simulink model "DC_Grid_New"  (R2022b)
settings: Solver=FixedStepAuto  StartTime=0.0  StopTime=48  FixedStep=0.01  RelTol=1e-3
undefined symbols (not defined in the file): C, cableLV, cableMV, flexible_load_autumn_shifted, flexible_load_spring_shifted, flexible_load_summer_shifted, flexible_load_winter_shifted, LowLoadP, LV, MV, PeakShP, Scaling_factor, Wind_scalefactor
libraries: DC_GRIDSIM_LIB x80, simulink x12
settings Model: Creator=mingreico  LastModifiedBy=mingreico

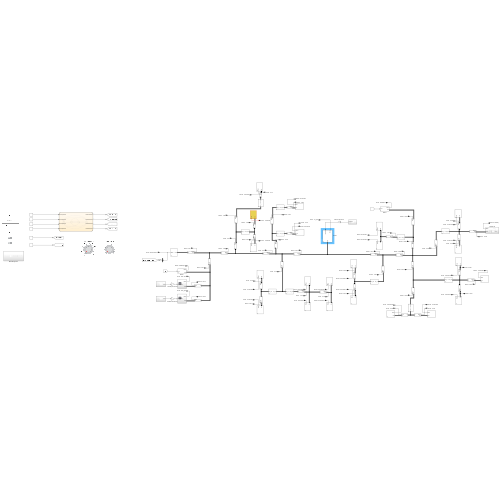
[thumbnail: Simulink's stored preview of the top-level diagram]
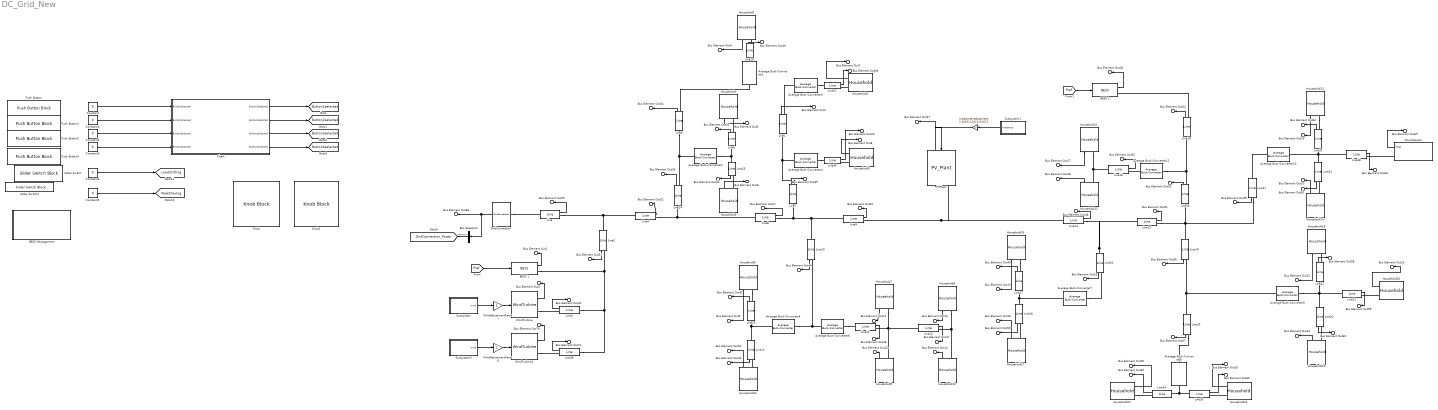
== system DC_Grid_New ==
  Average Buck-Converter{1..10,12} (11 alike) : DC_GRIDSIM_LIB/Average Buck-Converter  C=C  D=LV/MV
      settings: SourceProductName=DC GRIDSIM Library
  BESS 1 : DC_GRIDSIM_LIB/BESS  V_Bat=MV  Qbat=10000  SOC_init=0.5  SOC_min=0.1  SOC_max=0.9  P_max=10000
      settings: SourceProductName=DC GRIDSIM Library
  BESS 2 : DC_GRIDSIM_LIB/BESS  V_Bat=MV  Qbat=10000  SOC_init=0.5  SOC_min=0.1  SOC_max=0.9  P_max=10000
      settings: SourceProductName=DC GRIDSIM Library
  BESS Management : Subsystem
  Bus Selector2 : BusSelector  OutputSignals=Power
  Chart : Stateflow chart  TreatAsAtomicUnit=on
  Constant{,1..3} (4 alike) : Constant  Value=0  OutDataTypeStr=boolean
  Constant4 : Constant  Value=0
  Constant5 : Constant  Value=0
  FlexibleLoad : Subsystem
  GridConnection : DC_GRIDSIM_LIB/GridConnection  MV_Ref=MV
      settings: SourceProductName=DC GRIDSIM Library
  Household1 : DC_GRIDSIM_LIB/Household  ProfileSpring=Household4_Springallday  ProfileSummer=Household4_Summerallday  ProfileAutumn=Household4_Autumnallday  ProfileWinter=Household4_Winterallday  Timevector=Allday_timevector  k=Scaling_factor  VnomLoad=LV
      settings: SourceProductName=DC GRIDSIM Library
  Household10 : DC_GRIDSIM_LIB/Household  ProfileSpring=Household15_Springallday  ProfileSummer=Household15_Summerallday  ProfileAutumn=Household15_Autumnallday  ProfileWinter=Household15_Winterallday  Timevector=Allday_timevector  k=Scaling_factor  VnomLoad=LV
      settings: SourceProductName=DC GRIDSIM Library
  Household11 : DC_GRIDSIM_LIB/Household  ProfileSpring=Household26_Springallday  ProfileSummer=Household26_Summerallday  ProfileAutumn=Household26_Autumnallday  ProfileWinter=Household26_Winterallday  Timevector=Allday_timevector  k=Scaling_factor  VnomLoad=LV
      settings: SourceProductName=DC GRIDSIM Library
  Household12 : DC_GRIDSIM_LIB/Household  ProfileSpring=Household8_Springallday  ProfileSummer=Household8_Summerallday  ProfileAutumn=Household8_Autumnallday  ProfileWinter=Household8_Winterallday  Timevector=Allday_timevector  k=Scaling_factor  VnomLoad=LV
      settings: SourceProductName=DC GRIDSIM Library
  Household13 : DC_GRIDSIM_LIB/Household  ProfileSpring=Household9_Springallday  ProfileSummer=Household9_Summerallday  ProfileAutumn=Household9_Autumnallday  ProfileWinter=Household9_Winterallday  Timevector=Allday_timevector  k=Scaling_factor  VnomLoad=LV
      settings: SourceProductName=DC GRIDSIM Library
  Household14 : DC_GRIDSIM_LIB/Household  ProfileSpring=Household12_Springallday  ProfileSummer=Household12_Summerallday  ProfileAutumn=Household12_Autumnallday  ProfileWinter=Household12_Winterallday  Timevector=Allday_timevector  k=Scaling_factor  VnomLoad=LV
      settings: SourceProductName=DC GRIDSIM Library
  Household16 : DC_GRIDSIM_LIB/Household  ProfileSpring=Household11_Springallday  ProfileSummer=Household11_Summerallday  ProfileAutumn=Household11_Autumnallday  ProfileWinter=Household11_Winterallday  Timevector=Allday_timevector  k=Scaling_factor  VnomLoad=LV
      settings: SourceProductName=DC GRIDSIM Library
  Household17 : DC_GRIDSIM_LIB/Household  ProfileSpring=Household12_Springallday  ProfileSummer=Household12_Summerallday  ProfileAutumn=Household12_Autumnallday  ProfileWinter=Household12_Winterallday  Timevector=Allday_timevector  k=Scaling_factor  VnomLoad=LV
      settings: SourceProductName=DC GRIDSIM Library
  Household18 : DC_GRIDSIM_LIB/Household  ProfileSpring=Household3_Springallday  ProfileSummer=Household3_Summerallday  ProfileAutumn=Household3_Autumnallday  ProfileWinter=Household3_Winterallday  Timevector=Allday_timevector  k=Scaling_factor  VnomLoad=LV
      settings: SourceProductName=DC GRIDSIM Library
  Household19 : DC_GRIDSIM_LIB/Household  ProfileSpring=Household7_Springallday  ProfileSummer=Household7_Summerallday  ProfileAutumn=Household7_Autumnallday  ProfileWinter=Household7_Winterallday  Timevector=Allday_timevector  k=Scaling_factor  VnomLoad=LV
      settings: SourceProductName=DC GRIDSIM Library
  Household2 : DC_GRIDSIM_LIB/Household  ProfileSpring=Household3_Springallday  ProfileSummer=Household3_Summerallday  ProfileAutumn=Household3_Autumnallday  ProfileWinter=Household3_Winterallday  Timevector=Allday_timevector  k=Scaling_factor  VnomLoad=LV
      settings: SourceProductName=DC GRIDSIM Library
  Household20 : DC_GRIDSIM_LIB/Household  ProfileSpring=Household8_Springallday  ProfileSummer=Household8_Summerallday  ProfileAutumn=Household8_Autumnallday  ProfileWinter=Household8_Winterallday  Timevector=Allday_timevector  k=Scaling_factor  VnomLoad=LV
      settings: SourceProductName=DC GRIDSIM Library
  Household21 : DC_GRIDSIM_LIB/Household  ProfileSpring=Household10_Springallday  ProfileSummer=Household10_Summerallday  ProfileAutumn=Household10_Autumnallday  ProfileWinter=Household10_Winterallday  Timevector=Allday_timevector  k=Scaling_factor  VnomLoad=LV
      settings: SourceProductName=DC GRIDSIM Library
  Household22 : DC_GRIDSIM_LIB/Household  ProfileSpring=Household26_Springallday  ProfileSummer=Household26_Summerallday  ProfileAutumn=Household26_Autumnallday  ProfileWinter=Household26_Winterallday  Timevector=Allday_timevector  k=Scaling_factor  VnomLoad=LV
      settings: SourceProductName=DC GRIDSIM Library
  Household23 : DC_GRIDSIM_LIB/Household  ProfileSpring=Household33_Springallday  ProfileSummer=Household33_Summerallday  ProfileAutumn=Household33_Autumnallday  ProfileWinter=Household33_Winterallday  Timevector=Allday_timevector  k=Scaling_factor  VnomLoad=LV
      settings: SourceProductName=DC GRIDSIM Library
  Household3 : DC_GRIDSIM_LIB/Household  ProfileSpring=Household5_Springallday  ProfileSummer=Household5_Summerallday  ProfileAutumn=Household5_Autumnallday  ProfileWinter=Household5_Winterallday  Timevector=Allday_timevector  k=Scaling_factor  VnomLoad=LV
      settings: SourceProductName=DC GRIDSIM Library
  Household4 : DC_GRIDSIM_LIB/Household  ProfileSpring=Household7_Springallday  ProfileSummer=Household7_Summerallday  ProfileAutumn=Household7_Autumnallday  ProfileWinter=Household7_Winterallday  Timevector=Allday_timevector  k=Scaling_factor  VnomLoad=LV
      settings: SourceProductName=DC GRIDSIM Library
  Household5 : DC_GRIDSIM_LIB/Household  ProfileSpring=Household8_Springallday  ProfileSummer=Household8_Summerallday  ProfileAutumn=Household8_Autumnallday  ProfileWinter=Household8_Winterallday  Timevector=Allday_timevector  k=Scaling_factor  VnomLoad=LV
      settings: SourceProductName=DC GRIDSIM Library
  Household6 : DC_GRIDSIM_LIB/Household  ProfileSpring=Household9_Springallday  ProfileSummer=Household9_Summerallday  ProfileAutumn=Household9_Autumnallday  ProfileWinter=Household9_Winterallday  Timevector=Allday_timevector  k=Scaling_factor  VnomLoad=LV
      settings: SourceProductName=DC GRIDSIM Library
  Household7 : DC_GRIDSIM_LIB/Household  ProfileSpring=Household11_Springallday  ProfileSummer=Household11_Summerallday  ProfileAutumn=Household11_Autumnallday  ProfileWinter=Household11_Winterallday  Timevector=Allday_timevector  k=Scaling_factor  VnomLoad=LV
      settings: SourceProductName=DC GRIDSIM Library
  Household8 : DC_GRIDSIM_LIB/Household  ProfileSpring=Household14_Springallday  ProfileSummer=Household14_Summerallday  ProfileAutumn=Household14_Autumnallday  ProfileWinter=Household14_Winterallday  Timevector=Allday_timevector  k=Scaling_factor  VnomLoad=LV
      settings: SourceProductName=DC GRIDSIM Library
  Household9 : DC_GRIDSIM_LIB/Household  ProfileSpring=Household12_Springallday  ProfileSummer=Household12_Summerallday  ProfileAutumn=Household12_Autumnallday  ProfileWinter=Household12_Winterallday  Timevector=Allday_timevector  k=Scaling_factor  VnomLoad=LV
      settings: SourceProductName=DC GRIDSIM Library
  "Irradiance-adjustment " : Gain  Gain=0.9883216814160616
  Knob : KnobBlock  ScaleMin=0.9  ScaleMax=3  TickInterval=0.1
  Knob1 : KnobBlock  ScaleMin=0.9  ScaleMax=3  TickInterval=0.1
  Line : DC_GRIDSIM_LIB/Line  rho=rhoMV  l=1.4e3  A=cableMV
      settings: SourceProductName=DC GRIDSIM Library
  Line{1,4,7,14} (4 alike) : DC_GRIDSIM_LIB/Line  rho=rhoMV  l=1.3e3  A=cableMV
      settings: SourceProductName=DC GRIDSIM Library
  Line{5,8,10,17,24,30} (6 alike) : DC_GRIDSIM_LIB/Line  rho=rhoMV  l=1e3  A=cableMV
      settings: SourceProductName=DC GRIDSIM Library
  Line{6,11,13,21,25,27,38} (7 alike) : DC_GRIDSIM_LIB/Line  rho=rhoLV  l=50  A=cableLV
      settings: SourceProductName=DC GRIDSIM Library
  Line{12,23,31,33,36} (5 alike) : DC_GRIDSIM_LIB/Line  rho=rhoLV  l=35  A=cableLV
      settings: SourceProductName=DC GRIDSIM Library
  Line15 : DC_GRIDSIM_LIB/Line  rho=rhoMV  l=0.5e3  A=cableMV
      settings: SourceProductName=DC GRIDSIM Library
  Line16 : DC_GRIDSIM_LIB/Line  rho=rhoLV  l=10  A=cableLV
      settings: SourceProductName=DC GRIDSIM Library
  Line18 : DC_GRIDSIM_LIB/Line  rho=rhoMV  l=1.2e3  A=cableMV
      settings: SourceProductName=DC GRIDSIM Library
  Line19 : DC_GRIDSIM_LIB/Line  rho=rhoMV  l=0.6e3  A=cableMV
      settings: SourceProductName=DC GRIDSIM Library
  Line2 : DC_GRIDSIM_LIB/Line  rho=rhoMV  l=0.3e3  A=cableMV
      settings: SourceProductName=DC GRIDSIM Library
  Line20 : DC_GRIDSIM_LIB/Line  rho=rhoLV  l=45  A=cableLV
      settings: SourceProductName=DC GRIDSIM Library
  Line22 : DC_GRIDSIM_LIB/Line  rho=rhoLV  l=45  A=cableLV
      settings: SourceProductName=DC GRIDSIM Library
  Line26 : DC_GRIDSIM_LIB/Line  rho=1.68e-8  l=1.0  A=240e-6
      settings: SourceProductName=DC GRIDSIM Library
  Line28 : DC_GRIDSIM_LIB/Line  rho=rhoLV  l=60  A=cableLV
      settings: SourceProductName=DC GRIDSIM Library
  Line29 : DC_GRIDSIM_LIB/Line  rho=rhoMV  l=0.4e3  A=cableMV
      settings: SourceProductName=DC GRIDSIM Library
  Line3 : DC_GRIDSIM_LIB/Line  rho=rhoMV  l=0.3e3  A=cableMV
      settings: SourceProductName=DC GRIDSIM Library
  Line32 : DC_GRIDSIM_LIB/Line  rho=rhoLV  l=0.5e3  A=cableLV
      settings: SourceProductName=DC GRIDSIM Library
  Line34 : DC_GRIDSIM_LIB/Line  rho=rhoLV  l=70  A=cableLV
      settings: SourceProductName=DC GRIDSIM Library
  Line35 : DC_GRIDSIM_LIB/Line  rho=rhoLV  l=70  A=cableLV
      settings: SourceProductName=DC GRIDSIM Library
  Line37 : DC_GRIDSIM_LIB/Line  rho=rhoLV  l=60  A=cableLV
      settings: SourceProductName=DC GRIDSIM Library
  Line39 : DC_GRIDSIM_LIB/Line  rho=rhoMV  l=0.3e3  A=cableMV
      settings: SourceProductName=DC GRIDSIM Library
  Line9 : DC_GRIDSIM_LIB/Line  rho=rhoMV  l=2e3  A=cableMV
      settings: SourceProductName=DC GRIDSIM Library
  PVPlant : DC_GRIDSIM_LIB/PV_Plant  f_tilt=1.1  P_mpp=260e3  PR=0.8
      settings: SourceProductName=DC GRIDSIM Library
  Push Button : PushButtonBlock  ButtonText=Button_SpringAllday  OffValue=0.000000
  Push Button1 : PushButtonBlock  ButtonText=Button_SummerAllday  OffValue=0.000000
  Push Button2 : PushButtonBlock  ButtonText=Button_AutumnAllday  OffValue=0.000000
  Push Button3 : PushButtonBlock  ButtonText=Button_WinterAllday  OffValue=0.000000
  Slider Switch : SliderSwitchBlock  LabelPosition=Hide
      settings: Values={{'NOShift', 'FlexibleLoad_Shifted'}, [0 1]}
  Slider Switch1 : SliderSwitchBlock  LabelPosition=Hide
      settings: Values={{'NoPeakShaving', 'Peakshaved'}, [0 1]}
  Subsystem : Subsystem
  Subsystem1 : Subsystem
  Subsystem2 : Subsystem
  WindAdjustmentFactor : Gain
  WindAdjustmentFactor1 : Gain
  WindTurbine : DC_GRIDSIM_LIB/WindTurbine  SystemSampleTime=-1  VariantActivationTime=update diagram  Latency=0  AutoFrameSizeCalculation=off
      link override Blade radius: Value=28
      settings: SourceProductName=DC GRIDSIM Library
  WindTurbine1 : DC_GRIDSIM_LIB/WindTurbine  SystemSampleTime=-1  VariantActivationTime=update diagram  Latency=0  AutoFrameSizeCalculation=off
      link override Blade radius: Value=28
      settings: SourceProductName=DC GRIDSIM Library
  Bus Element Out38 : Outport  PortName=Results  Element=GridConnection
  Bus Element Out1 : Outport  PortName=Results  Element=GridBattery1
  Bus Element Out2 : Outport  PortName=Results  Element=Wind_gen1
  Bus Element Out4 : Outport  PortName=Results  Element=Household1
  Bus Element Out5 : Outport  PortName=Results  Element=Household2
  Bus Element Out6 : Outport  PortName=Results  Element=Household3
  Bus Element Out7 : Outport  PortName=Results  Element=Household4
  Bus Element Out8 : Outport  PortName=Results  Element=Household5
  Bus Element Out9 : Outport  PortName=Results  Element=Household6
  Bus Element Out10 : Outport  PortName=Results  Element=Household7
  Bus Element Out11 : Outport  PortName=Results  Element=Household8
  Bus Element Out12 : Outport  PortName=Results  Element=Household9
  Bus Element Out13 : Outport  PortName=Results  Element=Household10
  Bus Element Out14 : Outport  PortName=Results  Element=Household11
  Bus Element Out15 : Outport  PortName=Results  Element=Household12
  Bus Element Out16 : Outport  PortName=Results  Element=Household13
  Bus Element Out17 : Outport  PortName=Results  Element=Household14
  Bus Element Out18 : Outport  PortName=Results  Element=Household15
  Bus Element Out19 : Outport  PortName=Results  Element=Household16
  Bus Element Out20 : Outport  PortName=Results  Element=Household17
  Bus Element Out22 : Outport  PortName=Results  Element=Household19
  Bus Element Out23 : Outport  PortName=Results  Element=Household20
  Bus Element Out24 : Outport  PortName=Results  Element=Household21
  Bus Element Out25 : Outport  PortName=Results  Element=Household22
  Bus Element Out26 : Outport  PortName=Results  Element=Household23
  Bus Element Out27 : Outport  PortName=Results  Element=PV_gen1
  Bus Element Out28 : Outport  PortName=Results  Element=GridBattery2
  Bus Element Out29 : Outport  PortName=Results  Element=Line1
  Bus Element Out31 : Outport  PortName=Results  Element=Line3
  Bus Element Out32 : Outport  PortName=Results  Element=Line4
  Bus Element Out33 : Outport  PortName=Results  Element=Line5
  Bus Element Out34 : Outport  PortName=Results  Element=Line6
  Bus Element Out35 : Outport  PortName=Results  Element=Line7
  Bus Element Out36 : Outport  PortName=Results  Element=Line8
  Bus Element Out37 : Outport  PortName=Results  Element=Line9
  Bus Element Out39 : Outport  PortName=Results  Element=Line10
  Bus Element Out40 : Outport  PortName=Results  Element=Line11
  Bus Element Out41 : Outport  PortName=Results  Element=Line12
  Bus Element Out42 : Outport  PortName=Results  Element=Line13
  Bus Element Out43 : Outport  PortName=Results  Element=Line14
  Bus Element Out44 : Outport  PortName=Results  Element=Line15
  Bus Element Out45 : Outport  PortName=Results  Element=Line16
  Bus Element Out46 : Outport  PortName=Results  Element=Line17
  Bus Element Out47 : Outport  PortName=Results  Element=Line18
  Bus Element Out48 : Outport  PortName=Results  Element=Line19
  Bus Element Out49 : Outport  PortName=Results  Element=Line20
  Bus Element Out50 : Outport  PortName=Results  Element=Line21
  Bus Element Out51 : Outport  PortName=Results  Element=Line22
  Bus Element Out52 : Outport  PortName=Results  Element=Line23
  Bus Element Out53 : Outport  PortName=Results  Element=Line24
  Bus Element Out54 : Outport  PortName=Results  Element=Line25
  Bus Element Out55 : Outport  PortName=Results  Element=Line26
  Bus Element Out56 : Outport  PortName=Results  Element=Line27
  Bus Element Out57 : Outport  PortName=Results  Element=Line28
  Bus Element Out58 : Outport  PortName=Results  Element=Line29
  Bus Element Out59 : Outport  PortName=Results  Element=Line30
  Bus Element Out60 : Outport  PortName=Results  Element=Line31
  Bus Element Out61 : Outport  PortName=Results  Element=Line32
  Bus Element Out62 : Outport  PortName=Results  Element=Line33
  Bus Element Out64 : Outport  PortName=Results  Element=Line35
  Bus Element Out65 : Outport  PortName=Results  Element=Line36
  Bus Element Out21 : Outport  PortName=Results  Element=Line39
  Bus Element Out70 : Outport  PortName=Results  Element=Wind_gen2
  Bus Element Out71 : Outport  PortName=Results  Element=Line40
  Bus Element Out63 : Outport  PortName=Results  Element=Line34
  Bus Element Out69 : Outport  PortName=Results  Element=Flexibility
  Bus Element Out3 : Outport  PortName=Results  Element=Line2
  Bus Element Out30 : Outport  PortName=Results  Element=Line37
  Bus Element Out66 : Outport  PortName=Results  Element=Line38
  tag scope: Button1selected=global, Button2selected=global, Button3selected=global, Button4selected=global, GridConnection_Power=global, LoadShifting=global, PeakShaving=global
  wires:
  Chart/1(" Button1selected") -> [Button1selected]
  Chart/4(" Button4selected") -> [Button4selected]
  Chart/2(" Button2selected") -> [Button2selected]
  Constant1/1 -> Chart/2(Button2pressed)
  Chart/3(" Button3selected") -> [Button3selected]
  Constant4/1 -> [LoadShifting]
  Constant/1 -> Chart/1(Button1pressed)
  Constant3/1 -> Chart/4(Button4pressed)
  Constant5/1 -> [PeakShaving]
  Constant2/1 -> Chart/3(Button3pressed)
  [Pref] -> BESS 1/1
  BESS 1/1 -> Bus Element Out1/1
  Subsystem/1(wind) -> WindAdjustmentFactor/1
  WindAdjustmentFactor/1 -> WindTurbine/1
  WindTurbine/1 -> Bus Element Out2/1
  Household2/1 -> Bus Element Out4/1
  Household1/1 -> Bus Element Out5/1
  Household3/1 -> Bus Element Out6/1
  Household4/1 -> Bus Element Out7/1
  Household5/1 -> Bus Element Out8/1
  Household6/1 -> Bus Element Out9/1
  Household21/1 -> Bus Element Out10/1
  Household7/1 -> Bus Element Out11/1
  Household9/1 -> Bus Element Out12/1
  Household8/1 -> Bus Element Out13/1
  Household10/1 -> Bus Element Out14/1
  Household16/1 -> Bus Element Out15/1
  Household17/1 -> Bus Element Out16/1
  Household11/1 -> Bus Element Out17/1
  Household12/1 -> Bus Element Out18/1
  Household13/1 -> Bus Element Out19/1
  Household14/1 -> Bus Element Out20/1
  Household18/1 -> Bus Element Out22/1
  Household20/1 -> Bus Element Out23/1
  Household19/1 -> Bus Element Out24/1
  Household22/1 -> Bus Element Out25/1
  Household23/1 -> Bus Element Out26/1
  Subsystem1/1(irradiance) -> "Irradiance-adjustment "/1
  "Irradiance-adjustment "/1 -> PVPlant/1
  PVPlant/1 -> Bus Element Out27/1
  Bus Selector2/1 -> [GridConnection_Power]  "<Power>"
  GridConnection/1 -> Bus Element Out38/1, Bus Selector2/1
  [Pref] -> BESS 2/1
  BESS 2/1 -> Bus Element Out28/1
  Line/1 -> Bus Element Out29/1
  Line2/1 -> Bus Element Out31/1
  Line4/1 -> Bus Element Out32/1
  Line24/1 -> Bus Element Out33/1
  Line5/1 -> Bus Element Out34/1
  Line6/1 -> Bus Element Out35/1
  Line25/1 -> Bus Element Out36/1
  Line8/1 -> Bus Element Out37/1
  Line7/1 -> Bus Element Out39/1
  Line26/1 -> Bus Element Out40/1
  Line3/1 -> Bus Element Out41/1
  Line23/1 -> Bus Element Out42/1
  Line12/1 -> Bus Element Out43/1
  Line10/1 -> Bus Element Out44/1
  Line9/1 -> Bus Element Out45/1
  Line11/1 -> Bus Element Out46/1
  Line13/1 -> Bus Element Out47/1
  Line14/1 -> Bus Element Out48/1
  Line27/1 -> Bus Element Out49/1
  Line28/1 -> Bus Element Out50/1
  Line15/1 -> Bus Element Out51/1
  Line16/1 -> Bus Element Out52/1
  Line30/1 -> Bus Element Out53/1
  Line18/1 -> Bus Element Out54/1
  Line17/1 -> Bus Element Out55/1
  Line19/1 -> Bus Element Out56/1
  Line29/1 -> Bus Element Out57/1
  Line21/1 -> Bus Element Out58/1
  Line22/1 -> Bus Element Out59/1
  Line20/1 -> Bus Element Out60/1
  Line31/1 -> Bus Element Out61/1
  Line33/1 -> Bus Element Out62/1
  Line35/1 -> Bus Element Out65/1
  Line34/1 -> Bus Element Out64/1
  Line32/1 -> Bus Element Out21/1
  Line39/1 -> Bus Element Out71/1
  WindTurbine1/1 -> Bus Element Out70/1
  WindAdjustmentFactor1/1 -> WindTurbine1/1
  Subsystem2/1(wind) -> WindAdjustmentFactor1/1
  FlexibleLoad/1(Meas) -> Bus Element Out69/1
  Line38/1 -> Bus Element Out63/1
  Line1/1 -> Bus Element Out3/1
  Line36/1 -> Bus Element Out30/1
  Line37/1 -> Bus Element Out66/1
  connections:
  Line5/LConn1 -- Line24/RConn1 -- Average Buck-Converter2/LConn1
  Household12/RConn1 -- Household11/RConn1 -- Line16/LConn1
  GridConnection/LConn1 -- Line/LConn1
  WindTurbine/RConn1 -- Line3/RConn1
  Line3/LConn1 -- Line39/LConn1 -- BESS 1/RConn1 -- Line2/RConn1
  Line2/LConn1 -- Line/RConn1 -- Line4/LConn1
  Line5/RConn1 -- Average Buck-Converter1/LConn1
  Average Buck-Converter7/LConn1 -- Line32/RConn1
  Household3/RConn1 -- Line25/RConn1
  Line1/LConn1 -- Average Buck-Converter4/LConn1 -- Line7/RConn1
  Line4/RConn1 -- Line8/LConn1 -- Line24/LConn1
  Line8/RConn1 -- Line10/LConn1 -- Line9/LConn1 -- Line7/LConn1
  Household9/RConn1 -- Line13/LConn1 -- Household7/RConn1 -- Line11/RConn1
  Average Buck-Converter6/RConn1 -- Line11/LConn1
  Household10/RConn1 -- Household8/RConn1 -- Line13/RConn1
  Line9/RConn1 -- PVPlant/RConn1 -- Line14/LConn1
  Line20/LConn1 -- Average Buck-Converter9/RConn1 -- Line21/LConn1 -- Line22/LConn1
  Line15/RConn1 -- Line30/LConn1 -- Line19/LConn1 -- Line17/RConn1
  Household23/RConn1 -- Line35/RConn1
  Household18/RConn1 -- Line21/RConn1
  Household20/RConn1 -- Line22/RConn1
  Household19/RConn1 -- Line20/RConn1
  Average Buck-Converter1/RConn1 -- Line26/LConn1
  Household5/RConn1 -- Line36/RConn1
  Household4/RConn1 -- Line37/RConn1
  Household1/RConn1 -- Line6/RConn1
  Line25/LConn1 -- Average Buck-Converter2/RConn1 -- Line6/LConn1
  Household2/RConn1 -- Line26/RConn1
  Household6/RConn1 -- Line23/RConn1
  Household21/RConn1 -- Line12/RConn1
  Line23/LConn1 -- Average Buck-Converter5/RConn1 -- Line12/LConn1
  Average Buck-Converter6/LConn1 -- Average Buck-Converter5/LConn1 -- Line10/RConn1
  Household16/RConn1 -- Line27/RConn1
  Household17/RConn1 -- Line28/RConn1
  Line27/LConn1 -- Average Buck-Converter7/RConn1 -- Line28/LConn1
  Line19/RConn1 -- Average Buck-Converter9/LConn1 -- Line29/LConn1
  Line29/RConn1 -- Average Buck-Converter8/LConn1
  Line38/LConn1 -- Average Buck-Converter10/RConn1 -- Line33/LConn1 -- Line31/LConn1
  Average Buck-Converter10/LConn1 -- Line17/LConn1
  Line18/RConn1 -- BESS 2/RConn1
  Line30/RConn1 -- Average Buck-Converter12/LConn1 -- Line18/LConn1
  Household14/RConn1 -- Line31/RConn1
  Household13/RConn1 -- Line33/RConn1
  Household22/RConn1 -- Line34/RConn1
  Line34/LConn1 -- Line35/LConn1 -- Average Buck-Converter8/RConn1
  Line32/LConn1 -- Line15/LConn1 -- Line14/RConn1
  WindTurbine1/RConn1 -- Line39/RConn1
  FlexibleLoad/RConn1 -- Line38/RConn1
  Line1/RConn1 -- Average Buck-Converter3/LConn1
  Average Buck-Converter4/RConn1 -- Line36/LConn1
  Average Buck-Converter3/RConn1 -- Line37/LConn1
  Average Buck-Converter12/RConn1 -- Line16/RConn1

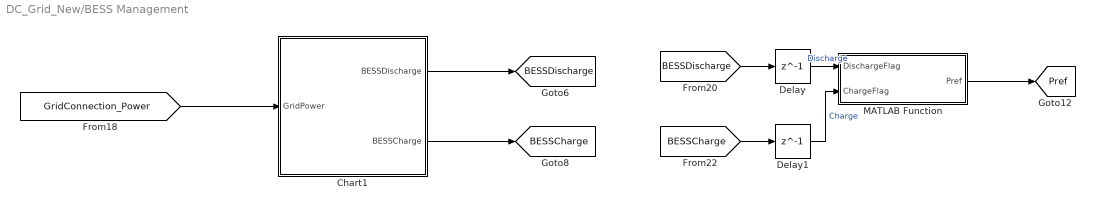
== system DC_Grid_New/BESS Management ==
  Chart1 : Stateflow chart  TreatAsAtomicUnit=on
  Delay : Delay  DelayLength=1
  Delay1 : Delay  DelayLength=1
  MATLAB Function : MATLAB Function  TreatAsAtomicUnit=on
  tag scope: BESSCharge=global, BESSDischarge=global, Pref=global
  wires:
  Delay1/1 -> MATLAB Function/2(ChargeFlag)  "Charge"
  Delay/1 -> MATLAB Function/1(DischargeFlag)  "Discharge"
  [BESSCharge] -> Delay1/1
  [GridConnection_Power] -> Chart1/1(GridPower)
  Chart1/1(BESSDischarge) -> [BESSDischarge]
  Chart1/2(BESSCharge) -> [BESSCharge]
  MATLAB Function/1(Pref) -> [Pref]
  [BESSDischarge] -> Delay/1

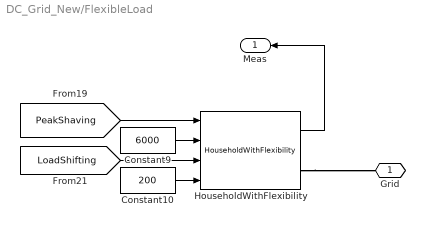
== system DC_Grid_New/FlexibleLoad ==
  Constant10 : Constant  Value=200
  Constant9 : Constant  Value=6000
  HouseholdWithFlexibility : DC_GRIDSIM_LIB/HouseholdWithFlexibility  Profile_spring=flexible_load_spring_shifted*10  Profile_summer=flexible_load_summer_shifted*10  Profile_autumn=flexible_load_autumn_shifted*10  Profile_winter=flexible_load_winter_shifted*10  Timevector=Allday_timevector  k=1  Vload=380  Base=800  flxQuota=0.5
      settings: SourceProductName=DC GRIDSIM Library
  Grid : PMIOPort  Side=Right
  Meas : Outport
  wires:
  Constant9/1 -> HouseholdWithFlexibility/2
  [LoadShifting] -> HouseholdWithFlexibility/3
  HouseholdWithFlexibility/1 -> Meas/1
  [PeakShaving] -> HouseholdWithFlexibility/1
  Constant10/1 -> HouseholdWithFlexibility/4
  connections:
  HouseholdWithFlexibility/RConn1 -- Grid/RConn1

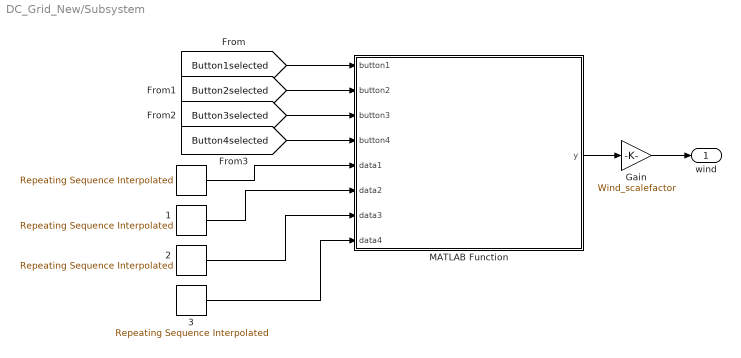
== system DC_Grid_New/Subsystem ==
  "  " : simulink/Sources/Repeating Sequence Interpolated  OutValues=Wind_SpringAllday  TimeValues=Allday_timevector  LookUpMeth=Interpolation-Use End Values  tsamp=0.01  OutMin=[]  OutMax=[]  OutDataTypeStr=double  OutputDataTypeScalingMode=double  OutDataType=fixdt(0,8)  OutScaling=2^-10
  "  1" : simulink/Sources/Repeating Sequence Interpolated  OutValues=Wind_SummerAllday  TimeValues=Allday_timevector  LookUpMeth=Interpolation-Use End Values  tsamp=0.01  OutMin=[]  OutMax=[]  OutDataTypeStr=double  OutputDataTypeScalingMode=double  OutDataType=fixdt(0,8)  OutScaling=2^-10
  "  2" : simulink/Sources/Repeating Sequence Interpolated  OutValues=Wind_AutumnAllday  TimeValues=Allday_timevector  LookUpMeth=Interpolation-Use End Values  tsamp=0.01  OutMin=[]  OutMax=[]  OutDataTypeStr=double  OutputDataTypeScalingMode=double  OutDataType=fixdt(0,8)  OutScaling=2^-10
  "  3" : simulink/Sources/Repeating Sequence Interpolated  OutValues=Wind_WinterAllday  TimeValues=Allday_timevector  LookUpMeth=Interpolation-Use End Values  tsamp=0.01  OutMin=[]  OutMax=[]  OutDataTypeStr=double  OutputDataTypeScalingMode=double  OutDataType=fixdt(0,8)  OutScaling=2^-10
  Gain : Gain  Gain=Wind_scalefactor
  MATLAB Function : MATLAB Function  TreatAsAtomicUnit=on
  wind : Outport
  wires:
  "  3"/1 -> MATLAB Function/8(data4)
  "  1"/1 -> MATLAB Function/6(data2)
  MATLAB Function/1(y) -> Gain/1
  "  "/1 -> MATLAB Function/5(data1)
  [Button2selected] -> MATLAB Function/2(button2)
  [Button4selected] -> MATLAB Function/4(button4)
  [Button3selected] -> MATLAB Function/3(button3)
  "  2"/1 -> MATLAB Function/7(data3)
  [Button1selected] -> MATLAB Function/1(button1)
  Gain/1 -> wind/1

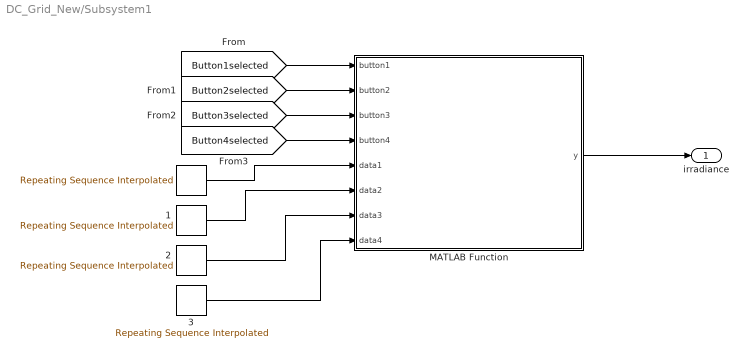
== system DC_Grid_New/Subsystem1 ==
  "  " : simulink/Sources/Repeating Sequence Interpolated  OutValues=Irradiance_SpringAllday  TimeValues=Allday_timevector  LookUpMeth=Interpolation-Use End Values  tsamp=0.01  OutMin=[]  OutMax=[]  OutDataTypeStr=double  OutputDataTypeScalingMode=double  OutDataType=fixdt(0,8)  OutScaling=2^-10
  "  1" : simulink/Sources/Repeating Sequence Interpolated  OutValues=Irradiance_SummerAllday  TimeValues=Allday_timevector  LookUpMeth=Interpolation-Use End Values  tsamp=0.01  OutMin=[]  OutMax=[]  OutDataTypeStr=double  OutputDataTypeScalingMode=double  OutDataType=fixdt(0,8)  OutScaling=2^-10
  "  2" : simulink/Sources/Repeating Sequence Interpolated  OutValues=Irradiance_AutumnAllday  TimeValues=Allday_timevector  LookUpMeth=Interpolation-Use End Values  tsamp=0.01  OutMin=[]  OutMax=[]  OutDataTypeStr=double  OutputDataTypeScalingMode=double  OutDataType=fixdt(0,8)  OutScaling=2^-10
  "  3" : simulink/Sources/Repeating Sequence Interpolated  OutValues=Irradiance_WinterAllday  TimeValues=Allday_timevector  LookUpMeth=Interpolation-Use End Values  tsamp=0.01  OutMin=[]  OutMax=[]  OutDataTypeStr=double  OutputDataTypeScalingMode=double  OutDataType=fixdt(0,8)  OutScaling=2^-10
  MATLAB Function : MATLAB Function  TreatAsAtomicUnit=on
  irradiance : Outport
  wires:
  "  3"/1 -> MATLAB Function/8(data4)
  "  1"/1 -> MATLAB Function/6(data2)
  [Button1selected] -> MATLAB Function/1(button1)
  "  2"/1 -> MATLAB Function/7(data3)
  [Button3selected] -> MATLAB Function/3(button3)
  [Button4selected] -> MATLAB Function/4(button4)
  [Button2selected] -> MATLAB Function/2(button2)
  "  "/1 -> MATLAB Function/5(data1)
  MATLAB Function/1(y) -> irradiance/1

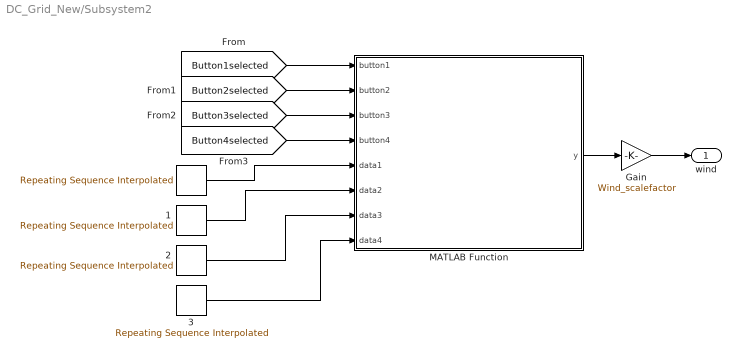
== system DC_Grid_New/Subsystem2 ==
  "  " : simulink/Sources/Repeating Sequence Interpolated  OutValues=Wind_SpringAllday  TimeValues=Allday_timevector  LookUpMeth=Interpolation-Use End Values  tsamp=0.01  OutMin=[]  OutMax=[]  OutDataTypeStr=double  OutputDataTypeScalingMode=double  OutDataType=fixdt(0,8)  OutScaling=2^-10
  "  1" : simulink/Sources/Repeating Sequence Interpolated  OutValues=Wind_SummerAllday  TimeValues=Allday_timevector  LookUpMeth=Interpolation-Use End Values  tsamp=0.01  OutMin=[]  OutMax=[]  OutDataTypeStr=double  OutputDataTypeScalingMode=double  OutDataType=fixdt(0,8)  OutScaling=2^-10
  "  2" : simulink/Sources/Repeating Sequence Interpolated  OutValues=Wind_AutumnAllday  TimeValues=Allday_timevector  LookUpMeth=Interpolation-Use End Values  tsamp=0.01  OutMin=[]  OutMax=[]  OutDataTypeStr=double  OutputDataTypeScalingMode=double  OutDataType=fixdt(0,8)  OutScaling=2^-10
  "  3" : simulink/Sources/Repeating Sequence Interpolated  OutValues=Wind_WinterAllday  TimeValues=Allday_timevector  LookUpMeth=Interpolation-Use End Values  tsamp=0.01  OutMin=[]  OutMax=[]  OutDataTypeStr=double  OutputDataTypeScalingMode=double  OutDataType=fixdt(0,8)  OutScaling=2^-10
  Gain : Gain  Gain=Wind_scalefactor
  MATLAB Function : MATLAB Function  TreatAsAtomicUnit=on
  wind : Outport
  wires:
  Gain/1 -> wind/1
  [Button1selected] -> MATLAB Function/1(button1)
  "  2"/1 -> MATLAB Function/7(data3)
  [Button3selected] -> MATLAB Function/3(button3)
  [Button4selected] -> MATLAB Function/4(button4)
  [Button2selected] -> MATLAB Function/2(button2)
  "  "/1 -> MATLAB Function/5(data1)
  MATLAB Function/1(y) -> Gain/1
  "  1"/1 -> MATLAB Function/6(data2)
  "  3"/1 -> MATLAB Function/8(data4)

== matlab function DC_Grid_New/Subsystem2/MATLAB Function ==
  data: button1 input; button2 input; button3 input; button4 input; data1 input; data2 input; y output; data3 input; data4 input
function y = fcn(button1, button2, button3, button4, data1,data2,data3, data4)
    if button1
        y = data1;
    elseif button2
        y =data2;
    elseif button3
        y = data3;
    elseif button4
        y = data4;
    else 
        y = data1;
    end
end

== matlab function DC_Grid_New/Subsystem1/MATLAB Function ==
  data: button1 input; button2 input; button3 input; button4 input; data1 input; data2 input; y output; data3 input; data4 input
function y = fcn(button1, button2, button3, button4, data1,data2,data3, data4)
    if button1
        y = data1;
    elseif button2
        y =data2;
    elseif button3
        y = data3;
    elseif button4
        y = data4;
    else 
        y = data1;
    end
end

== matlab function DC_Grid_New/BESS Management/MATLAB Function ==
  data: DischargeFlag input; Pref output; ChargeFlag input
function Pref = fcn(DischargeFlag, ChargeFlag)
    if ChargeFlag == 1
        Pref = 10000;
    elseif DischargeFlag == 1
         Pref = -5000;
    elseif ChargeFlag == 0 && DischargeFlag == 0
        Pref = 0;
    else 
        Pref = 0;
    end

== matlab function DC_Grid_New/Subsystem/MATLAB Function ==
  data: button1 input; button2 input; button3 input; button4 input; data1 input; data2 input; y output; data3 input; data4 input
function y = fcn(button1, button2, button3, button4, data1,data2,data3, data4)
    if button1
        y = data1;
    elseif button2
        y =data2;
    elseif button3
        y = data3;
    elseif button4
        y = data4;
    else 
        y = data1;
    end
end

== stateflow chart DC_Grid_New/BESS Management/Chart1 ==
  state Initial_Mode
    entry:
    BESSDischarge=0;
    BESSCharge=0;
    exit:
    BESSDischarge=0;
    BESSCharge=0;
  state Mode1_NormalLoading
    entry:
    BESSDischarge=0;
    BESSCharge=0;
    exit:
    BESSDischarge=0;
    BESSCharge=0;
  state Mode3_BESSCharging
    entry:
    BESSDischarge=0;
    BESSCharge=1;
    exit:
    BESSDischarge=0;
    BESSCharge=0;
  state Mode2_PeakShaving
    entry:
    BESSDischarge=1;
    BESSCharge=0;
    exit:
    BESSDischarge=0;
    BESSCharge=0;
  Mode1_NormalLoading -> Mode3_BESSCharging [order 1] : [duration (GridPower<LowLoadP)>1]
  (default) -> Initial_Mode
  Initial_Mode -> Mode1_NormalLoading : [after(1,sec)]
  Mode3_BESSCharging -> Mode1_NormalLoading : [duration (GridPower>LowLoadP)>1]
  Mode2_PeakShaving -> Mode1_NormalLoading : [duration(GridPower<PeakShP)>1]
  Mode1_NormalLoading -> Mode2_PeakShaving [order 2] : [duration (GridPower>PeakShP)>1]
  data: GridPower input; BESSDischarge output; BESSCharge output; LowLoadP parameter; PeakShP parameter

== stateflow chart DC_Grid_New/Chart ==
  settings: executeAtInitialization=1
  state Button1selected
  state Button2selected
  state Button3selected
  state Button4selected
  Button1selected -> Button4selected [order 4] : [Button4pressed]
  Button2selected -> Button4selected [order 4] : [Button4pressed]
  Button1selected -> Button3selected [order 3] : [Button3pressed]
  (default) -> Button1selected
  Button3selected -> Button4selected [order 2] : [Button4pressed]
  Button2selected -> Button3selected [order 2] : [Button3pressed]
  Button1selected -> Button1selected [order 2] : [Button1pressed]
  Button3selected -> Button2selected [order 1] : [Button2pressed]
  Button4selected -> Button4selected [order 2] : [Button4pressed]
  Button1selected -> Button2selected [order 1] : [Button2pressed]
  Button4selected -> Button3selected [order 1] : [Button3pressed]
  Button2selected -> Button1selected [order 1] : [Button1pressed]
  Button3selected -> Button3selected [order 3] : [Button3pressed]
  Button3selected -> Button1selected [order 4] : [Button1pressed]
  Button4selected -> Button1selected [order 3] : [Button1pressed]
  Button2selected -> Button2selected [order 3] : [Button2pressed]
  Button4selected -> Button2selected [order 4] : [Button2pressed]
  data: Button1selected output boolean; Button2selected output boolean; Button3selected output boolean; Button1pressed input boolean size=1; Button2pressed input boolean size=1; Button3pressed input boolean size=1; Button4pressed input boolean size=1; Button4selected output boolean
